simulink model "MoreElectricAircraftEMSHIL"  (R2023a)
settings: Solver=FixedStepAuto  StartTime=0.0  StopTime=350  RelTol=1e-3  EnableMultiTasking=on
PreLoadFcn:
  | Ts=100e-6;
InitFcn:
  | Ts=100e-6;
undefined symbols (not defined in the file): DiscIntNeverNeededParam, getfullname, IO682, Ion, Lithium
libraries: spsCurrentMeasurementLib x21, spsSeriesRLCBranchLib x19, spsVoltageMeasurementLib x19, speedgoatlib_IO682 x14, spsDiodeLib x10, spsControlledCurrentSourceLib x8, simulink x8, spsControlledVoltageSourceLib x7, spsIdealSwitchLib x6, spsThreePhaseParallelRLCLoadLib x1, spsPLL3phLib x1, spsThreePhaseVIMeasurementLib x1
(part 2 of 4)

== system MoreElectricAircraftEMSHIL/Hybrid Electric Aicraft System/Hybrid Electric Aicraft Plant/FC DC//DC Boost Converter ==
  VH* : Inport
  IL*(max) : Inport  Port=2
  Constant : Constant  Value=60
  DC/DC Boost Converter : Subsystem  mask(Average Value Boost DC/DC Converter){Inom=Inom, n=n, Tr=Tr, CL=CL}
      mask prompts: Inom "Full load current (A)"; n "Efficiency at Full and 10% load (%) [n1, n2]"; Tr "Response Time (s) (Voltage Regulator)"; CL "Load Capacitance (F)"
      mask help: This block implements an average-value DC/DC boost converter. Two inputs are provided for output voltage regulation and input current limitation
      mask init: same as MoreElectricAircraftEMSHIL/Hybrid Electric Aicraft System/Hybrid Electric Aicraft Plant/DC//DC Boost Converter/DC/DC Boost Converter
      mask DialogControl ParameterTabVar0 Prompt: Parameters
  DC/DC Buck Converter For DC bus precharge : Subsystem  mask(Average Value Buck DC/DC Converter){Inom=0.88*Inom, n=n, Tr=Tr, CL=CL}
      mask prompts: Inom "Full oad current (A)"; n "Efficiency @ Full and 10% load (%) [n1, n2]"; Tr "Response Time (s) (Voltage Regulator)"; CL "Load Capacitance (F)"
      mask help: This block implements an average-value DC/DC buck converter. Two inputs are provided for output voltage regulation and output current limitation
      mask init: same as MoreElectricAircraftEMSHIL/Hybrid Electric Aicraft System/Hybrid Electric Aicraft Plant/DC//DC Boost Converter/DC/DC Buck Converter For DC bus precharge
      mask DialogControl ParameterTabVar0 Prompt: Parameters
  +VH : PMIOPort  Side=Right
  +VL : PMIOPort  Port=2  Side=Left
  -VH : PMIOPort  Port=3  Side=Right
  -VL : PMIOPort  Port=4  Side=Left
  wires:
  [Iinbuck] -> DC/DC Boost Converter/3(Iinbuck)
  DC/DC Buck Converter For DC bus precharge/1(Iinbuck) -> [Iinbuck]
  Constant/1 -> DC/DC Buck Converter For DC bus precharge/1(VL*)
  VH*/1 -> DC/DC Boost Converter/1(VH*)
  IL*(max)/1 -> DC/DC Boost Converter/2(IL*(max)), DC/DC Buck Converter For DC bus precharge/2(IH*(max))
  connections:
  DC/DC Boost Converter/RConn2 -- -VH/RConn1 -- DC/DC Buck Converter For DC bus precharge/RConn2
  DC/DC Buck Converter For DC bus precharge/LConn2 -- -VL/RConn1 -- DC/DC Boost Converter/LConn2
  DC/DC Buck Converter For DC bus precharge/LConn1 -- +VL/RConn1 -- DC/DC Boost Converter/LConn1
  DC/DC Buck Converter For DC bus precharge/RConn1 -- +VH/RConn1 -- DC/DC Boost Converter/RConn1

== system MoreElectricAircraftEMSHIL/Hybrid Electric Aicraft System/Hybrid Electric Aicraft Plant/Fuel Cell Power Module (FCPM) ==
  Bus Selector : BusSelector  OutputSignals=Voltage,Current,Stack consumption (lpm) [Air(Yellow); Fuel(Magenta)],Flow Rate (lpm [Air(Yellow); Fuel(Magenta)]  OutputAsBus=on
  Contactors1 : Subsystem
  FCPM Controller : Subsystem
  Fuel Cell Stack : spsFuelCellStackLib/Fuel Cell Stack  PresetModel=No (User-Defined)  FcType=Proton Exchange Membrane (PEM)  Detailed=Detailed  Eoc="[52.5        52.46]"  NomVI="[250         41.15]"  EndVI="[320          39.2]"  Nc=65  n=50  TOp=45  AirFr=732  SuppPress="[1.16           1]"  Comp="[99.95           21            1]"  SignX=off  SignY=off  FlowRateH2=on  FlowRateAir=on  SystemTemp=off  SystemPH2=off  SystemPAir=off  FCDyn=on  FC_tau=1  Peak_O2=60  V_Under=2
      settings: LibrarySourceBlock=electricdrivelib/Extra Sources/Fuel Cell Stack
  Mux : Mux  Inputs=2
  Voltage Measurement : spsVoltageMeasurementLib/Voltage Measurement  PhasorSimulation=off  OutputType=Complex  PSBequivalent=0
  +VFC : PMIOPort  Side=Right
  -VFC : PMIOPort  Port=2  Side=Right
  Mesures : Outport  VectorParamsAs1DForOutWhenUnconnected=off
  Vfc : Outport  Port=2  VectorParamsAs1DForOutWhenUnconnected=off
  wires:
  FCPM Controller/3(H2Fr) -> Fuel Cell Stack/1
  FCPM Controller/2(AirFr) -> Fuel Cell Stack/2
  Fuel Cell Stack/1 -> FCPM Controller/1(IFC), Bus Selector/1
  FCPM Controller/1(IFCmax) -> Mux/1
  Bus Selector/1 -> Mux/2
  Mux/1 -> Mesures/1
  Voltage Measurement/1 -> Vfc/1
  connections:
  Contactors1/LConn1 -- Fuel Cell Stack/RConn1
  Voltage Measurement/LConn1 -- +VFC/RConn1 -- Contactors1/RConn1
  -VFC/RConn1 -- Fuel Cell Stack/RConn2 -- Voltage Measurement/LConn2

== system MoreElectricAircraftEMSHIL/Hybrid Electric Aicraft System/Hybrid Electric Aicraft Plant/Load Profile ==
  In1 : Inport
  1-D Lookup Table : Lookup_n-D  NumberOfTableDimensions=1  BreakpointsForDimension1="[0    20    30    35    40    45    50    60    70    90   125   130   140   160   170   180   190 210   220   230   235   245   250   260   270   300   310   320   330   340     350]"  Table="[0         0         0         0         0    5.8000    4.8000    4.8000   10.0000    9.4000  10.5000    5.0000    8.8000    7.0000    7.3000    2.5000    8.5000    7.5000    9.0000    8.9000 8.7000    0.7000    2.9000    2.3500    2.9000    2.9000    2.4000    2.9000    2.9000         0     0]"  InternalRulePriority=Speed  RndMeth=Simplest
  Aircraft Load(KVA) : Constant  Value=5.156351791530945
  Constant : Constant  Value=Ts
  Constant1 : Constant  Value=0
  Constant2 : Constant  Value=0.5
  Constant3 : Constant  Value=350
  Delay : Delay  DelayLength=1  InitialCondition=0
  Delay2 : Delay  DelayLength=1  InitialCondition=0
  Manual Load Control : Constant  Value=0
  Math Function : Math  Operator=mod
  Rate Transition : RateTransition  OutPortSampleTime=0.01
  Rate Transition1 : RateTransition
  Relational Operator : RelationalOperator  OutDataTypeStr=boolean  RndMeth=Simplest  InputSameDT=off
  Sum : Sum  Inputs=|++
  Sum1 : Sum  Inputs=|+-
  Switch : Switch  Criteria=u2 > Threshold  SaturateOnIntegerOverflow=off  InputSameDT=off
  Switch1 : Switch  Criteria=u2 > Threshold  Threshold=0.5  SaturateOnIntegerOverflow=off  InputSameDT=off
  Out1 : Outport
  wires:
  Constant1/1 -> Switch1/1
  Switch1/1 -> Math Function/1, Delay/1
  1-D Lookup Table/1 -> Switch/3
  Switch/1 -> Out1/1
  Constant/1 -> Sum/1
  Relational Operator/1 -> Switch1/2
  Sum/1 -> Switch1/3
  Constant2/1 -> Relational Operator/2
  Delay2/1 -> Sum1/2
  Aircraft Load(KVA)/1 -> Switch/1
  In1/1 -> Rate Transition/1
  Manual Load Control/1 -> Switch/2
  Delay/1 -> Sum/2
  Sum1/1 -> Rate Transition1/1
  Rate Transition/1 -> Delay2/1, Sum1/1
  Rate Transition1/1 -> Relational Operator/1
  Math Function/1 -> 1-D Lookup Table/1
  Constant3/1 -> Math Function/2

== system MoreElectricAircraftEMSHIL/Hybrid Electric Aicraft System/Hybrid Electric Aicraft Plant/Mesures 2 ==
  Current Measurement2 : spsCurrentMeasurementLib/Current Measurement  PhasorSimulation=off  OutputType=Complex  PSBequivalent=0
  Mux1 : Mux  Inputs=2
  Voltage Measurement2 : spsVoltageMeasurementLib/Voltage Measurement  PhasorSimulation=off  OutputType=Complex  PSBequivalent=0
  +M : PMIOPort  Side=Left
  O : PMIOPort  Port=2  Side=Right
  -M : PMIOPort  Port=3  Side=Left
  M : Outport  VectorParamsAs1DForOutWhenUnconnected=off
  wires:
  Voltage Measurement2/1 -> Mux1/2
  Current Measurement2/1 -> Mux1/1
  Mux1/1 -> M/1
  connections:
  +M/RConn1 -- Current Measurement2/LConn1
  -M/RConn1 -- Voltage Measurement2/LConn2
  Current Measurement2/RConn1 -- O/RConn1 -- Voltage Measurement2/LConn1

== system MoreElectricAircraftEMSHIL/Hybrid Electric Aicraft System/Hybrid Electric Aicraft Plant/Mesures1 ==
  Current Measurement2 : spsCurrentMeasurementLib/Current Measurement  PhasorSimulation=off  OutputType=Complex  PSBequivalent=0
  Mux1 : Mux  Inputs=2
  Voltage Measurement2 : spsVoltageMeasurementLib/Voltage Measurement  PhasorSimulation=off  OutputType=Complex  PSBequivalent=0
  +M : PMIOPort  Side=Left
  O : PMIOPort  Port=2  Side=Right
  -M : PMIOPort  Port=3  Side=Left
  M : Outport  VectorParamsAs1DForOutWhenUnconnected=off
  wires:
  Mux1/1 -> M/1
  Current Measurement2/1 -> Mux1/1
  Voltage Measurement2/1 -> Mux1/2
  connections:
  Voltage Measurement2/LConn1 -- O/RConn1 -- Current Measurement2/RConn1
  -M/RConn1 -- Voltage Measurement2/LConn2
  +M/RConn1 -- Current Measurement2/LConn1

== system MoreElectricAircraftEMSHIL/Hybrid Electric Aicraft System/Hybrid Electric Aicraft Plant/Protecting Resistor ==
  g : Inport
  Current Measurement : spsCurrentMeasurementLib/Current Measurement  PhasorSimulation=off  OutputType=Complex  PSBequivalent=0
  Ideal Switch : spsIdealSwitchLib/Ideal Switch  Ron=0.001  Lon=0  IC=0  Rs=10e3  Cs=inf  Measurements=off
  Mux : Mux  Inputs=2
  Series RLC Branch : spsSeriesRLCBranchLib/Series RLC Branch  LConnTagsString=__new0  RConnTagsString=__new0  BranchType=R  Resistance=6  Inductance=1e-3  SetiL0=off  InitialCurrent=0  Capacitance=1e-6  Setx0=off  InitialVoltage=0  Measurements=None
  Voltage Measurement : spsVoltageMeasurementLib/Voltage Measurement  PhasorSimulation=off  OutputType=Complex  PSBequivalent=0
  A : PMIOPort  Side=Right
  B : PMIOPort  Port=2  Side=Right
  Mesures : Outport  VectorParamsAs1DForOutWhenUnconnected=off
  wires:
  g/1 -> Ideal Switch/1
  Current Measurement/1 -> Mux/1
  Voltage Measurement/1 -> Mux/2
  Mux/1 -> Mesures/1
  connections:
  Series RLC Branch/LConn1 -- Ideal Switch/LConn1
  B/RConn1 -- Series RLC Branch/RConn1 -- Voltage Measurement/LConn2
  Current Measurement/RConn1 -- Ideal Switch/RConn1
  Current Measurement/LConn1 -- A/RConn1 -- Voltage Measurement/LConn1

== system MoreElectricAircraftEMSHIL/Hybrid Electric Aicraft System/Energy Management System/HIL/Plant Rx ==
  Bus Creator : BusCreator  Inputs=8
  "Decode v2 " : speedgoatlib_IO682/Decode v2   parMode=Standard  parLabel=[100 101 102 103 104 105 106 107]  parDataType=[1 1 1 1 1 1 1 1]  parResolution=[500 500 100 500 100 100 10 1]  parSyncMask=hex2dec('0x0')  parSyncValue=hex2dec('0x0')  parCustomDataType=Raw  parDataLSB=9  parDataMSB=31  parBitPosition=[9, 31]  parScaleBNR=1  parExponent=8  parMantissa=14  parTimeTags=off  parHoldLastVal=on  parStatus=off
      settings: SourceProductName=Simulink Real-Time: Speedgoat I/O Blockset
  Demux2 : Demux  Outputs=8
  Rate Transition4 : RateTransition  InitialCondition=1
  "Receive v3 " : speedgoatlib_IO682/Receive v3   parModuleId=1  parChannel=1  parMaxWords=50  parMinWords=1  parSampleTime=0.01
      settings: SourceProductName=Simulink Real-Time: Speedgoat I/O Blockset
  "Setup v3 " : speedgoatlib_IO682/Setup v3   parModuleId=1  parBoardVariant=IO682-4-4  parPciSlot=-1  parTimerCount=4000  parChannelMode=Manual  parInBitRate1=100000  parInBufferMode1=Individual  parInEnable1=on  parInParity1=on  parInInternalWrap1=off  parInBitRate2=100000  parInBufferMode2=Individual  parInEnable2=on  parInParity2=on  parInInternalWrap2=off  parInBitRate3=100000  parInBufferMode3=Individual  parInEnable3=on  parInParity3=on  parInInternalWrap3=off  parInBitRate4=100000  parInBufferMode4=Individual  parInEnable4=on  parInParity4=on  parInInternalWrap4=off  parInBitRate5=100000  parInBufferMode5=Individual  parInEnable5=on  parInParity5=on  parInInternalWrap5=off  parInBitRate6=100000  parInBufferMode6=Individual  parInEnable6=on  parInParity6=on  parInInternalWrap6=off  parInBitRate7=100000  parInBufferMode7=Individual  parInEnable7=on  parInParity7=on  parInInternalWrap7=off  parInBitRate8=100000  parInBufferMode8=Individual  parInEnable8=on  parInParity8=on  parInInternalWrap8=off  parInBitRate9=100000  parInBufferMode9=Individual  parInEnable9=on  parInParity9=on  parInInternalWrap9=off  parInBitRate10=100000  parInBufferMode10=Individual  parInEnable10=on  parInParity10=on  parInInternalWrap10=off  parInBitRate11=100000  parInBufferMode11=Individual  parInEnable11=on  parInParity11=on  parInInternalWrap11=off  parInBitRate12=100000  parInBufferMode12=Individual  parInEnable12=on  parInParity12=on  parInInternalWrap12=off  parInBitRate13=100000  parInBufferMode13=Individual  parInEnable13=on  parInParity13=on  parInInternalWrap13=off  parInBitRate14=100000  parInBufferMode14=Individual  parInEnable14=on  parInParity14=on  parInInternalWrap14=off  parInBitRate15=100000  parInBufferMode15=Individual  parInEnable15=on  parInParity15=on  parInInternalWrap15=off  parInBitRate16=100000  parInBufferMode16=Individual  parInEnable16=on  parInParity16=on  parInInternalWrap16=off  parOutBitRate1=100000  parOutParity1=Odd  parOutProtocolError1=None  parOutEnable1=on  parOutBitRate2=100000  parOutParity2=Odd  parOutProtocolError2=None  parOutEnable2=on  parOutBitRate3=100000  parOutParity3=Odd  parOutProtocolError3=None  parOutEnable3=on  parOutBitRate4=100000  parOutParity4=Odd  parOutProtocolError4=None  parOutEnable4=on  parOutBitRate5=100000  parOutParity5=Odd  parOutProtocolError5=None  parOutEnable5=on  parOutBitRate6=100000  parOutParity6=Odd  parOutProtocolError6=None  parOutEnable6=on  parOutBitRate7=100000  parOutParity7=Odd  parOutProtocolError7=None  parOutEnable7=on  parOutBitRate8=100000  parOutParity8=Odd  parOutProtocolError8=None  parOutEnable8=on  parOutBitRate9=100000  parOutParity9=Odd  parOutProtocolError9=None  parOutEnable9=on  parOutBitRate10=100000  parOutParity10=Odd  parOutProtocolError10=None  parOutEnable10=on  parOutBitRate11=100000  parOutParity11=Odd  parOutProtocolError11=None  parOutEnable11=on  parOutBitRate12=100000  parOutParity12=Odd  parOutProtocolError12=None  parOutEnable12=on  parOutBitRate13=100000  parOutParity13=Odd  parOutProtocolError13=None  parOutEnable13=on  parOutBitRate14=100000  parOutParity14=Odd  parOutProtocolError14=None  parOutEnable14=on  parOutBitRate15=100000  parOutParity15=Odd  parOutProtocolError15=None  parOutEnable15=on  parOutBitRate16=100000  parOutParity16=Odd  parOutProtocolError16=None  parOutEnable16=on  parChConfigFile=''  parScheduleMode=Manual  parScheduledMsgConfigFile=''  parHwDeviceId=hex2dec('0830')  parTimeSource=Internal timer  parChInConfig=[158 8 7 7 1;158 8 7 7 1;158 8 7 7 1;158 8 7 7 1]  parChOutConfig=[158 0 4 7;158 0 4 7;158 0 4 7;158 0 4 7]  parScheduledMessages=0  parIsSlrealtime=on
      settings: SourceProductName=Simulink Real-Time: Speedgoat I/O Blockset
  BusEMS : Outport
  wires:
  Rate Transition4/1 -> Demux2/1
  "Receive v3 "/1 -> "Decode v2 "/1
  "Decode v2 "/1 -> Rate Transition4/1
  Demux2/3 -> Bus Creator/3  "IBat_maxD"
  Demux2/7 -> Bus Creator/7  "Res_ON"
  Demux2/2 -> Bus Creator/2  "VDC1"
  Demux2/6 -> Bus Creator/6  "VBatt"
  Demux2/5 -> Bus Creator/5  "IBatt_maxC"
  Demux2/1 -> Bus Creator/1  "IFC_max"
  Demux2/8 -> Bus Creator/8  "Load_ON"
  Demux2/4 -> Bus Creator/4  "VDC2"
  Bus Creator/1 -> BusEMS/1

== system MoreElectricAircraftEMSHIL/Hybrid Electric Aicraft System/Energy Management System/HIL/Plant Tx ==
  BusPlant : Inport
  Bus Selector1 : BusSelector  OutputSignals=SOC (%),Current (A),Voltage (V)
  Bus Selector2 : BusSelector  OutputSignals=Current I,Voltage V,SOC %
  Bus Selector3 : BusSelector  OutputSignals=FuelCell,Battery,SC,IConvFCout,IConvBattout,Iinv,Vfc
  Encode v2 1 : speedgoatlib_IO682/Encode v2   parMode=Standard  parLabel=[300 301 302 303 304 305 306 307 310 311 312 313 314 315 316 317 320]  parDataType=[1 1 1 1 1 1 1 1 1 1 1 1 1 1 1 1 1]  parResolution=[300 100 300 300 100 700 100 100 100 100 100 300 100 100 100 100 100]  parBits=[19]  parSdi=[0]  parSsm=[-1]  parCustomDataType=Raw  parDataLSB=9  parDataMSB=31  parBitPosition=[9, 31]  parScaleBNR=1  parExponent=8  parMantissa=14  parEnSSM=off
      settings: SourceProductName=Simulink Real-Time: Speedgoat I/O Blockset
  Mux3 : Mux  Inputs=11
  Rate Transition : RateTransition
  Send v3 1 : speedgoatlib_IO682/Send v3   parModuleId=1  parChannel=2  parSampleTime=0.01
      settings: SourceProductName=Simulink Real-Time: Speedgoat I/O Blockset
  wires:
  Bus Selector2/1 -> Mux3/5  "<Current I>"
  Bus Selector1/1 -> Mux3/2  "<SOC (%)>"
  Bus Selector3/6 -> Mux3/10  "<Iinv>"
  Bus Selector3/4 -> Mux3/8  "<IConvFCout>"
  Bus Selector3/2 -> Bus Selector1/1  "<Battery>"
  Rate Transition/1 -> Send v3 1/1
  Bus Selector3/3 -> Bus Selector2/1  "<SC>"
  Bus Selector3/5 -> Mux3/9  "<IConvBattout>"
  Mux3/1 -> Encode v2 1/1
  Encode v2 1/1 -> Rate Transition/1
  Bus Selector3/1 -> Mux3/1  "<FuelCell>"
  BusPlant/1 -> Bus Selector3/1
  Bus Selector1/2 -> Mux3/3  "<Current (A)>"
  Bus Selector1/3 -> Mux3/4  "<Voltage (V)>"
  Bus Selector2/2 -> Mux3/6  "<Voltage V>"
  Bus Selector2/3 -> Mux3/7  "<SOC %>"
  Bus Selector3/7 -> Mux3/11  "<Vfc>"

== system MoreElectricAircraftEMSHIL/Hybrid Electric Aicraft System/Energy Management System/MIL/Battery DC//DC charge converter reference ==
  IBAT* : Inport
  Constant1 : Constant  Value=0
  Constant8 : Constant  Value=58
  Switch5 : Switch  Criteria=u2 > Threshold  SaturateOnIntegerOverflow=off  InputSameDT=off
  IBAT_maxC* : Outport  VectorParamsAs1DForOutWhenUnconnected=off
  VBAT* : Outport  Port=2  VectorParamsAs1DForOutWhenUnconnected=off
  wires:
  [EMSON] -> Switch5/2
  IBAT*/1 -> Switch5/1
  Constant1/1 -> Switch5/3
  Switch5/1 -> IBAT_maxC*/1
  Constant8/1 -> VBAT*/1

== system MoreElectricAircraftEMSHIL/Hybrid Electric Aicraft System/Energy Management System/MIL/Battery DC//DC discharge converter references  ==
  IBAT* : Inport
  Constant10 : Constant  Value=0
  Constant6 : Constant  Value=270
  Switch1 : Switch  Criteria=u2 > Threshold  SaturateOnIntegerOverflow=off  InputSameDT=off
  Switch10 : Switch  Criteria=u2 > Threshold  SaturateOnIntegerOverflow=off  InputSameDT=off
  IBAT_maxD* : Outport  VectorParamsAs1DForOutWhenUnconnected=off
  VDC2* : Outport  Port=2  VectorParamsAs1DForOutWhenUnconnected=off
  wires:
  Switch10/1 -> VDC2*/1
  [EMSON] -> Switch10/2
  Constant6/1 -> Switch10/3
  IBAT*/1 -> Switch1/1
  [Vdcref] -> Switch10/1
  [EMSON] -> Switch1/2
  Switch1/1 -> IBAT_maxD*/1
  Constant10/1 -> Switch1/3

== system MoreElectricAircraftEMSHIL/Hybrid Electric Aicraft System/Energy Management System/MIL/FC DC//DC converter references ==
  IFC* : Inport
  Add1 : Sum  Inputs=+-
  Constant11 : Constant  Value=212
  Constant22 : Constant  Value=270
  Constant3 : Constant  Value=15
  Constant4 : Constant  Value=297
  Constant7 : Constant  Value=250
  Fcn : Fcn  Expr=u(1)*(u(1)<u(2))+u(2)*(u(1)>=u(2))
  Mux6 : Mux  Inputs=2
  Relational Operator6 : RelationalOperator  Operator=<=  OutDataTypeStr=boolean  InputSameDT=off
  Switch : Switch  Criteria=u2 > Threshold  SaturateOnIntegerOverflow=off  InputSameDT=off
  Switch6 : Switch  Criteria=u2 > Threshold  SaturateOnIntegerOverflow=off  InputSameDT=off
  Switch9 : Switch  Criteria=u2 > Threshold  SaturateOnIntegerOverflow=off  InputSameDT=off
  filter : Subsystem
  IFC*max : Outport  VectorParamsAs1DForOutWhenUnconnected=off
  VDC1* : Outport  Port=2  VectorParamsAs1DForOutWhenUnconnected=off
  wires:
  [EMSON] -> Switch9/2
  Switch9/1 -> VDC1*/1
  Constant4/1 -> Switch9/1
  Constant22/1 -> Switch9/3
  Switch6/1 -> Switch/1
  Constant11/1 -> Relational Operator6/2, Switch6/3
  Relational Operator6/1 -> Switch6/2
  Constant7/1 -> Switch/3
  Constant3/1 -> Add1/2
  IFC*/1 -> Relational Operator6/1, Switch6/1
  Mux6/1 -> Fcn/1
  Fcn/1 -> filter/1(I)
  [EMSON] -> Switch/2
  Switch/1 -> Mux6/1
  filter/1(If) -> IFC*max/1
  Add1/1 -> Mux6/2
  [IFCAllow] -> Add1/1

== system MoreElectricAircraftEMSHIL/Hybrid Electric Aicraft System/Energy Management System/MIL/Load Disconnect ==
  SOC : Inport
  Vdc : Inport  Port=2
  Clock : Clock
  Constant1 : Constant  Value=0.1
  Constant18 : Constant  Value=0
  Constant19 : Constant  Value=0
  Constant2 : Constant  Value=270
  Constant5 : Constant
  Constant9 : Constant  Value=200
  Data Type Conversion2 : DataTypeConversion  SaturateOnIntegerOverflow=off  RndMeth=Floor
  Emergency_Landing : Constant
  Logical Operator : Logic  AllPortsSameDT=off  OutDataTypeStr=boolean
  Logical Operator3 : Logic  Inputs=3  AllPortsSameDT=off  OutDataTypeStr=boolean
  Relational Operator : RelationalOperator  OutDataTypeStr=boolean  InputSameDT=off
  Relational Operator1 : RelationalOperator  OutDataTypeStr=boolean  InputSameDT=off
  Relational Operator3 : RelationalOperator  Operator=<=  OutDataTypeStr=boolean  InputSameDT=off
  Relational Operator5 : RelationalOperator  Operator=<=  OutDataTypeStr=boolean  InputSameDT=off
  SOC_Low : Constant  Value=3
  Switch2 : Switch  Criteria=u2 > Threshold  SaturateOnIntegerOverflow=off  InputSameDT=off
  Switch7 : Switch  Criteria=u2 > Threshold  SaturateOnIntegerOverflow=off  InputSameDT=off
  Switch8 : Switch  Criteria=u2 > Threshold  SaturateOnIntegerOverflow=off  InputSameDT=off
  Unit Delay : UnitDelay  SampleTime=Ts  HasFrameUpgradeWarning=on
  Unit Delay4 : UnitDelay  InitialCondition=1  SampleTime=Ts  HasFrameUpgradeWarning=on
  LoadON : Outport  VectorParamsAs1DForOutWhenUnconnected=off
  tag scope: EMSON=global
  wires:
  Data Type Conversion2/1 -> LoadON/1  "Loadon"
  Relational Operator3/1 -> Switch8/2
  Constant18/1 -> Switch7/1
  Switch8/1 -> Switch2/3
  SOC_Low/1 -> Relational Operator5/2
  Switch7/1 -> Unit Delay4/1, Logical Operator3/1  "soc1"
  Unit Delay4/1 -> Switch7/3
  Unit Delay/1 -> Switch8/3
  SOC/1 -> Relational Operator5/1
  Logical Operator3/1 -> Data Type Conversion2/1
  Constant19/1 -> Switch8/1
  Constant9/1 -> Relational Operator3/2
  Relational Operator/1 -> Switch2/2
  Constant5/1 -> Switch2/1
  Constant2/1 -> Relational Operator/2
  Switch2/1 -> [EMSON], Unit Delay/1, Logical Operator3/2
  Vdc/1 -> Relational Operator/1, Relational Operator3/1
  Relational Operator5/1 -> Logical Operator/2  "Battery Health"
  Clock/1 -> Relational Operator1/1
  Constant1/1 -> Relational Operator1/2
  Relational Operator1/1 -> Logical Operator/1
  Logical Operator/1 -> Switch7/2
  Emergency_Landing/1 -> Logical Operator3/3

== system MoreElectricAircraftEMSHIL/Hybrid Electric Aicraft System/Energy Management System/MIL/Protecting resistor connect ==
  Vdc : Inport
  Constant12 : Constant  Value=290
  Constant13 : Constant
  Constant14 : Constant  Value=285
  Constant15 : Constant  Value=0
  Data Type Conversion1 : DataTypeConversion  SaturateOnIntegerOverflow=off  RndMeth=Floor
  Relational Operator1 : RelationalOperator  OutDataTypeStr=boolean  InputSameDT=off
  Relational Operator2 : RelationalOperator  Operator=<=  OutDataTypeStr=boolean  InputSameDT=off
  Switch3 : Switch  Criteria=u2 > Threshold  SaturateOnIntegerOverflow=off  InputSameDT=off
  Switch4 : Switch  Criteria=u2 > Threshold  SaturateOnIntegerOverflow=off  InputSameDT=off
  Unit Delay1 : UnitDelay  SampleTime=Ts  HasFrameUpgradeWarning=on
  ResON : Outport  VectorParamsAs1DForOutWhenUnconnected=off
  wires:
  Unit Delay1/1 -> Switch4/3
  Vdc/1 -> Relational Operator1/1, Relational Operator2/1
  Switch4/1 -> Switch3/3
  Switch3/1 -> Data Type Conversion1/1, Unit Delay1/1
  Relational Operator1/1 -> Switch3/2
  Relational Operator2/1 -> Switch4/2
  Data Type Conversion1/1 -> ResON/1
  Constant15/1 -> Switch4/1
  Constant13/1 -> Switch3/1
  Constant14/1 -> Relational Operator2/2
  Constant12/1 -> Relational Operator1/2

== system MoreElectricAircraftEMSHIL/Hybrid Electric Aicraft System/Energy Management System/MIL/Subsystem ==
  note: Max DC bus voltage
  note: Min DC bus voltage
  Pload : Inport
  SOC : Inport  Port=2
  Constant1 : Constant  Value=260
  Constant2 : Constant  Value=285
  Constant20 : Constant  Value=270
  Constant21 : Constant  Value=60
  Discrete PI Controller1 : Subsystem  DialogController=POWERSYS.PowerSysDialog  mask(Discrete PI Controller){Kp=10, Ki=10, Par_Limits=[140 0], Init=0, Ts=Ts}
      mask prompts: Kp "Proportional gain (Kp):"; Ki "Integral gain (Ki):"; Par_Limits "Output limits: [ Upper   Lower ]"; Init "Output initial value:"; Ts "Sample time:"
      mask help: This block implements a discrete PI controller.
      mask init:
      | UpperLimit=Par_Limits(1);
      | LowerLimit=Par_Limits(2);
      | power_initmask();
      mask Help: This block is part of a subset of blocks in the Extras library that does not have documentation associated with it, other than the block mask description.
      mask Display: disp('PI');
  Discrete PI Controller2 : Subsystem  DialogController=POWERSYS.PowerSysDialog  mask(Discrete PI Controller){Kp=50000, Ki=5000, Par_Limits=[3400 -1500], Init=0, Ts=200e-3}
      mask prompts: Kp "Proportional gain (Kp):"; Ki "Integral gain (Ki):"; Par_Limits "Output limits: [ Upper   Lower ]"; Init "Output initial value:"; Ts "Sample time:"
      mask help: This block implements a discrete PI controller.
      mask init:
      | UpperLimit=Par_Limits(1);
      | LowerLimit=Par_Limits(2);
      | power_initmask();
      mask Help: This block is part of a subset of blocks in the Extras library that does not have documentation associated with it, other than the block mask description.
      mask Display: disp('PI');
  Discrete PI Controller3 : Subsystem  DialogController=POWERSYS.PowerSysDialog  mask(Discrete PI Controller){Kp=10, Ki=10, Par_Limits=[0 -100], Init=0, Ts=Ts}
      mask prompts: Kp "Proportional gain (Kp):"; Ki "Integral gain (Ki):"; Par_Limits "Output limits: [ Upper   Lower ]"; Init "Output initial value:"; Ts "Sample time:"
      mask help: This block implements a discrete PI controller.
      mask init:
      | UpperLimit=Par_Limits(1);
      | LowerLimit=Par_Limits(2);
      | power_initmask();
      mask Help: This block is part of a subset of blocks in the Extras library that does not have documentation associated with it, other than the block mask description.
      mask Display: disp('PI');
  Discrete PI Controller4 : Subsystem  DialogController=POWERSYS.PowerSysDialog  mask(Discrete PI Controller){Kp=10, Ki=10, Par_Limits=[80 -20], Init=0, Ts=Ts}
      mask prompts: Kp "Proportional gain (Kp):"; Ki "Integral gain (Ki):"; Par_Limits "Output limits: [ Upper   Lower ]"; Init "Output initial value:"; Ts "Sample time:"
      mask help: This block implements a discrete PI controller.
      mask init:
      | UpperLimit=Par_Limits(1);
      | LowerLimit=Par_Limits(2);
      | power_initmask();
      mask Help: This block is part of a subset of blocks in the Extras library that does not have documentation associated with it, other than the block mask description.
      mask Display: disp('PI');
  Divide : Product  Inputs=*/
  Gain : Gain  Gain=-1
  Gain2 : Gain  Gain=1/0.85
  Saturation : Saturate  UpperLimit=inf  LowerLimit=0.01
  Saturation1 : Saturate  UpperLimit=80  LowerLimit=0
  Saturation2 : Saturate  UpperLimit=20  LowerLimit=0
  Saturation3 : Saturate  UpperLimit=8800  LowerLimit=850
  Saturation4 : Saturate  UpperLimit=250  LowerLimit=20
  Sum : Sum  Inputs=|+-
  Sum1 : Sum  Inputs=|-+
  Sum2 : Sum  Inputs=|-+
  Sum3 : Sum  Inputs=|+-
  Sum4 : Sum  Inputs=|++
  Sum5 : Sum  Inputs=|+-
  Sum6 : Sum  Inputs=|++
  filter2 : Subsystem
  IFC* : Outport  VectorParamsAs1DForOutWhenUnconnected=off
  IBATD* : Outport  Port=2  VectorParamsAs1DForOutWhenUnconnected=off
  IBATC* : Outport  Port=3  VectorParamsAs1DForOutWhenUnconnected=off
  tag scope: Vdcref=scoped
  wires:
  Divide/1 -> Sum4/1
  Discrete PI Controller1/1(Out) -> Sum4/2
  filter2/1(If) -> IBATC*/1
  Constant20/1 -> Sum/1, [Vdcref]
  SOC/1 -> Sum1/2
  Saturation3/1 -> Gain2/1
  Saturation/1 -> Divide/2
  Saturation1/1 -> IBATD*/1
  Constant1/1 -> Sum3/1
  Discrete PI Controller2/1(Out) -> Sum2/1
  Sum5/1 -> Discrete PI Controller3/1(Error)
  Sum4/1 -> Sum6/1
  Constant21/1 -> Sum1/1
  Pload/1 -> Sum2/2
  Gain2/1 -> Divide/1
  Sum6/1 -> Saturation4/1
  Saturation4/1 -> IFC*/1
  Constant2/1 -> Sum5/1
  Sum3/1 -> Discrete PI Controller1/1(Error)
  Gain/1 -> Saturation2/1
  Discrete PI Controller4/1(Out) -> Saturation1/1, Gain/1
  Sum2/1 -> Saturation3/1
  Sum1/1 -> Discrete PI Controller2/1(Error)
  Saturation2/1 -> filter2/1(I)
  [Vdc] -> Sum5/2
  [Vdc] -> Sum/2
  Discrete PI Controller3/1(Out) -> Sum6/2
  [Vdc] -> Sum3/2
  [S_Vfc] -> Saturation/1
  Sum/1 -> Discrete PI Controller4/1(Error)

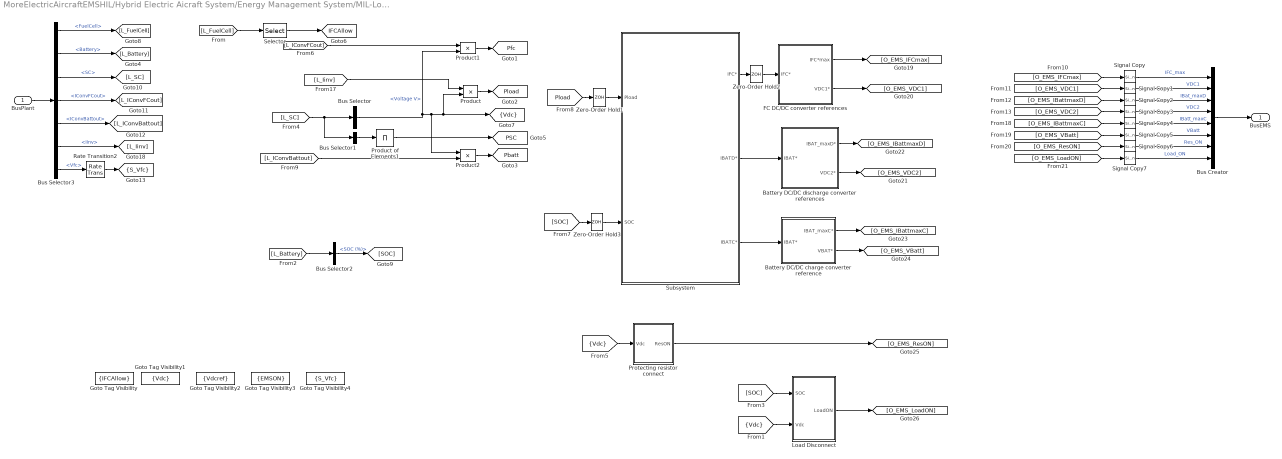
== system MoreElectricAircraftEMSHIL/Hybrid Electric Aicraft System/Energy Management System/MIL-Loopback/EMS ==
  BusPlant : Inport
  Battery DC/DC charge converter reference : Subsystem
  "Battery DC/DC discharge converter references " : Subsystem
  Bus Creator : BusCreator  Inputs=8
  Bus Selector : BusSelector  OutputSignals=Voltage V
  Bus Selector1 : BusSelector  OutputSignals=Current I,Voltage V  OutputAsBus=on
  Bus Selector2 : BusSelector  OutputSignals=SOC (%)
  Bus Selector3 : BusSelector  OutputSignals=FuelCell,Battery,SC,IConvFCout,IConvBattout,Iinv,Vfc
  FC DC/DC converter references : Subsystem
  Goto Tag Visibility : GotoTagVisibility  GotoTag=IFCAllow
  Goto Tag Visibility1 : GotoTagVisibility  GotoTag=Vdc
  Goto Tag Visibility2 : GotoTagVisibility  GotoTag=Vdcref
  Goto Tag Visibility3 : GotoTagVisibility  GotoTag=EMSON
  Goto Tag Visibility4 : GotoTagVisibility  GotoTag=S_Vfc
  Load Disconnect : Subsystem
  Product : Product  RndMeth=Zero
  Product of Elements1 : Product  Inputs=*
  Product1 : Product  RndMeth=Zero
  Product2 : Product  RndMeth=Zero
  Protecting resistor connect : Subsystem
  Rate Transition2 : RateTransition  InitialCondition=1
  Selector : Selector  InputPortWidth=7  IndexOptions=Index vector (dialog)  Indices=1  OutputSizes=1
  Signal Copy{,1..7} (8 alike) : SignalConversion  OverrideOpt=off
  Subsystem : Subsystem
  Zero-Order Hold1 : ZeroOrderHold  SampleTime=200e-3
  Zero-Order Hold2 : ZeroOrderHold  SampleTime=200e-3
  Zero-Order Hold3 : ZeroOrderHold  SampleTime=200e-3
  BusEMS : Outport  VectorParamsAs1DForOutWhenUnconnected=off
  tag scope: IFCAllow=global, PSC=global, Pbatt=global, Pfc=global, Pload=global, S_Vfc=scoped, Vdc=scoped
  wires:
  Bus Selector/1 -> Product1/2, Product2/1, Product/2, [Vdc]  "<Voltage V>"
  [L_IConvFCout] -> Product1/1
  [L_IConvBattout] -> Product2/2
  [L_Iinv] -> Product/1
  [L_SC] -> Bus Selector/1, Bus Selector1/1
  Product/1 -> [Pload]
  Product1/1 -> [Pfc]
  Product2/1 -> [Pbatt]
  Bus Selector1/1 -> Product of Elements1/1
  Product of Elements1/1 -> [PSC]
  Selector/1 -> [IFCAllow]
  [L_Battery] -> Bus Selector2/1
  Bus Selector2/1 -> [SOC]  "<SOC (%)>"
  [SOC] -> Load Disconnect/1(SOC)
  [Vdc] -> Load Disconnect/2(Vdc)
  [Vdc] -> Protecting resistor connect/1(Vdc)
  Subsystem/1(IFC*) -> Zero-Order Hold2/1
  [Pload] -> Zero-Order Hold1/1
  [SOC] -> Zero-Order Hold3/1
  Zero-Order Hold2/1 -> FC DC/DC converter references/1(IFC*)
  Subsystem/2(IBATD*) -> "Battery DC/DC discharge converter references "/1(IBAT*)
  Subsystem/3(IBATC*) -> Battery DC/DC charge converter reference/1(IBAT*)
  Zero-Order Hold1/1 -> Subsystem/1(Pload)
  Zero-Order Hold3/1 -> Subsystem/2(SOC)
  FC DC/DC converter references/1(IFC*max) -> [O_EMS_IFCmax]
  FC DC/DC converter references/2(VDC1*) -> [O_EMS_VDC1]
  "Battery DC/DC discharge converter references "/1(IBAT_maxD*) -> [O_EMS_IBattmaxD]
  "Battery DC/DC discharge converter references "/2(VDC2*) -> [O_EMS_VDC2]
  Battery DC/DC charge converter reference/1(IBAT_maxC*) -> [O_EMS_IBattmaxC]
  Battery DC/DC charge converter reference/2(VBAT*) -> [O_EMS_VBatt]
  Protecting resistor connect/1(ResON) -> [O_EMS_ResON]
  Load Disconnect/1(LoadON) -> [O_EMS_LoadON]
  BusPlant/1 -> Bus Selector3/1
  Bus Selector3/1 -> [L_FuelCell]  "<FuelCell>"
  Bus Selector3/2 -> [L_Battery]  "<Battery>"
  Bus Selector3/3 -> [L_SC]  "<SC>"
  Bus Selector3/4 -> [L_IConvFCout]  "<IConvFCout>"
  Bus Selector3/5 -> [L_IConvBattout]  "<IConvBattout>"
  Bus Selector3/6 -> [L_Iinv]  "<Iinv>"
  [L_FuelCell] -> Selector/1
  [O_EMS_IFCmax] -> Signal Copy/1
  [O_EMS_VDC1] -> Signal Copy1/1
  [O_EMS_IBattmaxD] -> Signal Copy2/1
  [O_EMS_VDC2] -> Signal Copy3/1
  [O_EMS_IBattmaxC] -> Signal Copy4/1
  [O_EMS_VBatt] -> Signal Copy5/1
  [O_EMS_ResON] -> Signal Copy6/1
  [O_EMS_LoadON] -> Signal Copy7/1
  Signal Copy1/1 -> Bus Creator/2  "VDC1"
  Signal Copy2/1 -> Bus Creator/3  "IBat_maxD"
  Signal Copy3/1 -> Bus Creator/4  "VDC2"
  Signal Copy4/1 -> Bus Creator/5  "IBatt_maxC"
  Signal Copy5/1 -> Bus Creator/6  "VBatt"
  Signal Copy6/1 -> Bus Creator/7  "Res_ON"
  Signal Copy7/1 -> Bus Creator/8  "Load_ON"
  Signal Copy/1 -> Bus Creator/1  "IFC_max"
  Bus Creator/1 -> BusEMS/1
  Bus Selector3/7 -> Rate Transition2/1  "<Vfc>"
  Rate Transition2/1 -> [S_Vfc]

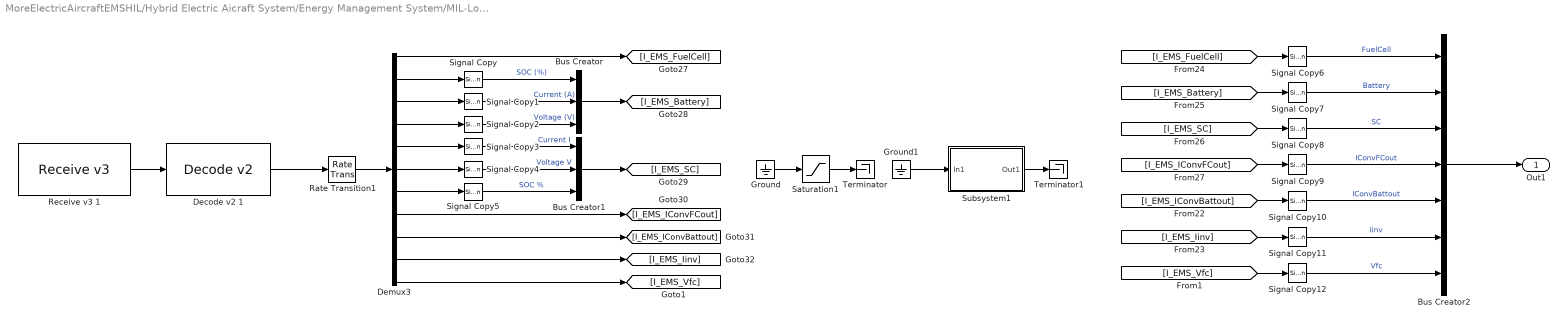
== system MoreElectricAircraftEMSHIL/Hybrid Electric Aicraft System/Energy Management System/MIL-Loopback/EMS Rx ==
  Bus Creator : BusCreator  Inputs=3
  Bus Creator1 : BusCreator  Inputs=3
  Bus Creator2 : BusCreator  Inputs=7
  Decode v2 1 : speedgoatlib_IO682/Decode v2   parMode=Standard  parLabel=[300 301 302 303 304 305 306 307 310 311 312 313 314 315 316 317 320]  parDataType=[1 1 1 1 1 1 1 1 1 1 1 1 1 1 1 1 1]  parResolution=[300 100 300 300 100 700 100 100 100 100 100 300 100 100 100 100 100]  parSyncMask=hex2dec('0x0')  parSyncValue=hex2dec('0x0')  parCustomDataType=Raw  parDataLSB=9  parDataMSB=31  parBitPosition=[9, 31]  parScaleBNR=1  parExponent=8  parMantissa=14  parTimeTags=off  parHoldLastVal=on  parStatus=off
      settings: SourceProductName=Simulink Real-Time: Speedgoat I/O Blockset
  Demux3 : Demux  Outputs=11
  Ground : Ground
  Ground1 : Ground
  Rate Transition1 : RateTransition  InitialCondition=1
  Receive v3 1 : speedgoatlib_IO682/Receive v3   parModuleId=1  parChannel=2  parMaxWords=100  parMinWords=1  parSampleTime=0.01
      settings: SourceProductName=Simulink Real-Time: Speedgoat I/O Blockset
  Saturation1 : Saturate  UpperLimit=1000000000  LowerLimit=269
  Signal Copy{,1..12} (13 alike) : SignalConversion  OverrideOpt=off
  Subsystem1 : Subsystem
  Terminator : Terminator
  Terminator1 : Terminator
  Out1 : Outport
  wires:
  Subsystem1/1(Out1) -> Terminator1/1
  Ground/1 -> Saturation1/1
  Demux3/2 -> Signal Copy/1
  Rate Transition1/1 -> Demux3/1
  Demux3/1 -> [I_EMS_FuelCell]
  Signal Copy1/1 -> Bus Creator/2  "Current (A)"
  Signal Copy5/1 -> Bus Creator1/3  "SOC %"
  Bus Creator1/1 -> [I_EMS_SC]
  Demux3/9 -> [I_EMS_IConvBattout]
  Demux3/5 -> Signal Copy3/1
  Bus Creator/1 -> [I_EMS_Battery]
  Signal Copy4/1 -> Bus Creator1/2  "Voltage V"
  Demux3/7 -> Signal Copy5/1
  Signal Copy3/1 -> Bus Creator1/1  "Current I"
  Saturation1/1 -> Terminator/1
  Ground1/1 -> Subsystem1/1(In1)
  Demux3/6 -> Signal Copy4/1
  Demux3/4 -> Signal Copy2/1
  Decode v2 1/1 -> Rate Transition1/1
  Signal Copy2/1 -> Bus Creator/3  "Voltage (V)"
  Demux3/10 -> [I_EMS_Iinv]
  Demux3/3 -> Signal Copy1/1
  Receive v3 1/1 -> Decode v2 1/1
  Signal Copy/1 -> Bus Creator/1  "SOC (%)"
  Demux3/8 -> [I_EMS_IConvFCout]
  Bus Creator2/1 -> Out1/1
  Signal Copy9/1 -> Bus Creator2/4  "IConvFCout"
  Signal Copy8/1 -> Bus Creator2/3  "SC"
  Signal Copy10/1 -> Bus Creator2/5  "IConvBattout"
  [I_EMS_Battery] -> Signal Copy7/1
  Signal Copy11/1 -> Bus Creator2/6  "Iinv"
  [I_EMS_Iinv] -> Signal Copy11/1
  [I_EMS_SC] -> Signal Copy8/1
  [I_EMS_IConvBattout] -> Signal Copy10/1
  Signal Copy6/1 -> Bus Creator2/1  "FuelCell"
  Signal Copy7/1 -> Bus Creator2/2  "Battery"
  [I_EMS_IConvFCout] -> Signal Copy9/1
  [I_EMS_FuelCell] -> Signal Copy6/1
  Demux3/11 -> [I_EMS_Vfc]
  [I_EMS_Vfc] -> Signal Copy12/1
  Signal Copy12/1 -> Bus Creator2/7  "Vfc"

== system MoreElectricAircraftEMSHIL/Hybrid Electric Aicraft System/Energy Management System/MIL-Loopback/EMS Tx ==
  IFC*max1 : Inport
  Bus Selector3 : BusSelector  OutputSignals=IFC_max,VDC1,IBat_maxD,VDC2,IBatt_maxC,VBatt,Res_ON,Load_ON
  "Encode v2 " : speedgoatlib_IO682/Encode v2   parMode=Standard  parLabel=[100 101 102 103 104 105 106 107]  parDataType=[1 1 1 1 1 1 1 1]  parResolution=[500 500 100 500 100 100 10 1]  parBits=[19]  parSdi=[0]  parSsm=[-1]  parCustomDataType=Raw  parDataLSB=9  parDataMSB=31  parBitPosition=[9, 31]  parScaleBNR=1  parExponent=8  parMantissa=14  parEnSSM=off
      settings: SourceProductName=Simulink Real-Time: Speedgoat I/O Blockset
  Mux2 : Mux  Inputs=8
  Rate Transition3 : RateTransition
  "Send v3 " : speedgoatlib_IO682/Send v3   parModuleId=1  parChannel=1  parSampleTime=0.01
      settings: SourceProductName=Simulink Real-Time: Speedgoat I/O Blockset
  "Setup v3 " : speedgoatlib_IO682/Setup v3   parModuleId=1  parBoardVariant=IO682-4-4  parPciSlot=-1  parTimerCount=4000  parChannelMode=Manual  parInBitRate1=100000  parInBufferMode1=Individual  parInEnable1=on  parInParity1=on  parInInternalWrap1=off  parInBitRate2=100000  parInBufferMode2=Individual  parInEnable2=on  parInParity2=on  parInInternalWrap2=off  parInBitRate3=100000  parInBufferMode3=Individual  parInEnable3=on  parInParity3=on  parInInternalWrap3=off  parInBitRate4=100000  parInBufferMode4=Individual  parInEnable4=on  parInParity4=on  parInInternalWrap4=off  parInBitRate5=100000  parInBufferMode5=Individual  parInEnable5=on  parInParity5=on  parInInternalWrap5=off  parInBitRate6=100000  parInBufferMode6=Individual  parInEnable6=on  parInParity6=on  parInInternalWrap6=off  parInBitRate7=100000  parInBufferMode7=Individual  parInEnable7=on  parInParity7=on  parInInternalWrap7=off  parInBitRate8=100000  parInBufferMode8=Individual  parInEnable8=on  parInParity8=on  parInInternalWrap8=off  parInBitRate9=100000  parInBufferMode9=Individual  parInEnable9=on  parInParity9=on  parInInternalWrap9=off  parInBitRate10=100000  parInBufferMode10=Individual  parInEnable10=on  parInParity10=on  parInInternalWrap10=off  parInBitRate11=100000  parInBufferMode11=Individual  parInEnable11=on  parInParity11=on  parInInternalWrap11=off  parInBitRate12=100000  parInBufferMode12=Individual  parInEnable12=on  parInParity12=on  parInInternalWrap12=off  parInBitRate13=100000  parInBufferMode13=Individual  parInEnable13=on  parInParity13=on  parInInternalWrap13=off  parInBitRate14=100000  parInBufferMode14=Individual  parInEnable14=on  parInParity14=on  parInInternalWrap14=off  parInBitRate15=100000  parInBufferMode15=Individual  parInEnable15=on  parInParity15=on  parInInternalWrap15=off  parInBitRate16=100000  parInBufferMode16=Individual  parInEnable16=on  parInParity16=on  parInInternalWrap16=off  parOutBitRate1=100000  parOutParity1=Odd  parOutProtocolError1=None  parOutEnable1=on  parOutBitRate2=100000  parOutParity2=Odd  parOutProtocolError2=None  parOutEnable2=on  parOutBitRate3=100000  parOutParity3=Odd  parOutProtocolError3=None  parOutEnable3=on  parOutBitRate4=100000  parOutParity4=Odd  parOutProtocolError4=None  parOutEnable4=on  parOutBitRate5=100000  parOutParity5=Odd  parOutProtocolError5=None  parOutEnable5=on  parOutBitRate6=100000  parOutParity6=Odd  parOutProtocolError6=None  parOutEnable6=on  parOutBitRate7=100000  parOutParity7=Odd  parOutProtocolError7=None  parOutEnable7=on  parOutBitRate8=100000  parOutParity8=Odd  parOutProtocolError8=None  parOutEnable8=on  parOutBitRate9=100000  parOutParity9=Odd  parOutProtocolError9=None  parOutEnable9=on  parOutBitRate10=100000  parOutParity10=Odd  parOutProtocolError10=None  parOutEnable10=on  parOutBitRate11=100000  parOutParity11=Odd  parOutProtocolError11=None  parOutEnable11=on  parOutBitRate12=100000  parOutParity12=Odd  parOutProtocolError12=None  parOutEnable12=on  parOutBitRate13=100000  parOutParity13=Odd  parOutProtocolError13=None  parOutEnable13=on  parOutBitRate14=100000  parOutParity14=Odd  parOutProtocolError14=None  parOutEnable14=on  parOutBitRate15=100000  parOutParity15=Odd  parOutProtocolError15=None  parOutEnable15=on  parOutBitRate16=100000  parOutParity16=Odd  parOutProtocolError16=None  parOutEnable16=on  parChConfigFile=''  parScheduleMode=Manual  parScheduledMsgConfigFile=''  parHwDeviceId=hex2dec('0830')  parTimeSource=Internal timer  parChInConfig=[158 8 7 7 1;158 8 7 7 1;158 8 7 7 1;158 8 7 7 1]  parChOutConfig=[158 0 4 7;158 0 4 7;158 0 4 7;158 0 4 7]  parScheduledMessages=0  parIsSlrealtime=on
      settings: SourceProductName=Simulink Real-Time: Speedgoat I/O Blockset
  wires:
  "Encode v2 "/1 -> Rate Transition3/1
  Mux2/1 -> "Encode v2 "/1
  Rate Transition3/1 -> "Send v3 "/1
  IFC*max1/1 -> Bus Selector3/1
  Bus Selector3/1 -> Mux2/1  "<IFC_max>"
  Bus Selector3/2 -> Mux2/2  "<VDC1>"
  Bus Selector3/3 -> Mux2/3  "<IBat_maxD>"
  Bus Selector3/4 -> Mux2/4  "<VDC2>"
  Bus Selector3/5 -> Mux2/5  "<IBatt_maxC>"
  Bus Selector3/6 -> Mux2/6  "<VBatt>"
  Bus Selector3/7 -> Mux2/7  "<Res_ON>"
  Bus Selector3/8 -> Mux2/8  "<Load_ON>"

== system MoreElectricAircraftEMSHIL/Hybrid Electric Aicraft System/Energy Management System/MIL-Loopback/Plant Rx ==
  Bus Creator : BusCreator  Inputs=8
  "Decode v2 " : speedgoatlib_IO682/Decode v2   parMode=Standard  parLabel=[100 101 102 103 104 105 106 107]  parDataType=[1 1 1 1 1 1 1 1]  parResolution=[500 500 100 500 100 100 10 1]  parSyncMask=hex2dec('0x0')  parSyncValue=hex2dec('0x0')  parCustomDataType=Raw  parDataLSB=9  parDataMSB=31  parBitPosition=[9, 31]  parScaleBNR=1  parExponent=8  parMantissa=14  parTimeTags=off  parHoldLastVal=on  parStatus=off
      settings: SourceProductName=Simulink Real-Time: Speedgoat I/O Blockset
  Demux2 : Demux  Outputs=8
  Rate Transition4 : RateTransition  InitialCondition=1
  "Receive v3 " : speedgoatlib_IO682/Receive v3   parModuleId=1  parChannel=1  parMaxWords=50  parMinWords=1  parSampleTime=0.01
      settings: SourceProductName=Simulink Real-Time: Speedgoat I/O Blockset
  BusEMS : Outport
  wires:
  Rate Transition4/1 -> Demux2/1
  "Receive v3 "/1 -> "Decode v2 "/1
  "Decode v2 "/1 -> Rate Transition4/1
  Demux2/3 -> Bus Creator/3  "IBat_maxD"
  Demux2/7 -> Bus Creator/7  "Res_ON"
  Demux2/2 -> Bus Creator/2  "VDC1"
  Demux2/6 -> Bus Creator/6  "VBatt"
  Demux2/5 -> Bus Creator/5  "IBatt_maxC"
  Demux2/1 -> Bus Creator/1  "IFC_max"
  Demux2/8 -> Bus Creator/8  "Load_ON"
  Demux2/4 -> Bus Creator/4  "VDC2"
  Bus Creator/1 -> BusEMS/1

== system MoreElectricAircraftEMSHIL/Hybrid Electric Aicraft System/Energy Management System/MIL-Loopback/Plant Tx ==
  BusPlant : Inport
  Bus Selector1 : BusSelector  OutputSignals=SOC (%),Current (A),Voltage (V)
  Bus Selector2 : BusSelector  OutputSignals=Current I,Voltage V,SOC %
  Bus Selector3 : BusSelector  OutputSignals=FuelCell,Battery,SC,IConvFCout,IConvBattout,Iinv,Vfc
  Encode v2 1 : speedgoatlib_IO682/Encode v2   parMode=Standard  parLabel=[300 301 302 303 304 305 306 307 310 311 312 313 314 315 316 317 320]  parDataType=[1 1 1 1 1 1 1 1 1 1 1 1 1 1 1 1 1]  parResolution=[300 100 300 300 100 700 100 100 100 100 100 300 100 100 100 100 100]  parBits=[19]  parSdi=[0]  parSsm=[-1]  parCustomDataType=Raw  parDataLSB=9  parDataMSB=31  parBitPosition=[9, 31]  parScaleBNR=1  parExponent=8  parMantissa=14  parEnSSM=off
      settings: SourceProductName=Simulink Real-Time: Speedgoat I/O Blockset
  Mux3 : Mux  Inputs=11
  Rate Transition : RateTransition
  Send v3 1 : speedgoatlib_IO682/Send v3   parModuleId=1  parChannel=2  parSampleTime=0.01
      settings: SourceProductName=Simulink Real-Time: Speedgoat I/O Blockset
  wires:
  Bus Selector2/1 -> Mux3/5  "<Current I>"
  Bus Selector1/1 -> Mux3/2  "<SOC (%)>"
  Bus Selector3/6 -> Mux3/10  "<Iinv>"
  Bus Selector3/4 -> Mux3/8  "<IConvFCout>"
  Bus Selector3/2 -> Bus Selector1/1  "<Battery>"
  Rate Transition/1 -> Send v3 1/1
  Bus Selector3/3 -> Bus Selector2/1  "<SC>"
  Bus Selector3/5 -> Mux3/9  "<IConvBattout>"
  Mux3/1 -> Encode v2 1/1
  Encode v2 1/1 -> Rate Transition/1
  Bus Selector3/1 -> Mux3/1  "<FuelCell>"
  BusPlant/1 -> Bus Selector3/1
  Bus Selector1/2 -> Mux3/3  "<Current (A)>"
  Bus Selector1/3 -> Mux3/4  "<Voltage (V)>"
  Bus Selector2/2 -> Mux3/6  "<Voltage V>"
  Bus Selector2/3 -> Mux3/7  "<SOC %>"
  Bus Selector3/7 -> Mux3/11  "<Vfc>"

== system MoreElectricAircraftEMSHIL/Hybrid Electric Aicraft System/Hybrid Electric Aicraft Plant/3-phase AC load/Dynamic Impedance ==
  S : Inport
  pf : Inport  Port=2
  Fcn3 : Fcn  Expr=(sqrt(u(2)^2-u(1)^2))
  Fcn5 : Fcn  Expr=u(1)*u(2)
  Gain1 : Gain  Gain=2e3
  Gain3 : Gain  Gain=2e3
  Impedance Calculation : Subsystem
  Mux1 : Mux  Inputs=2
  Mux3 : Mux  Inputs=2
  Real-Imag to Complex1 : RealImagToComplex
  Z : Outport  VectorParamsAs1DForOutWhenUnconnected=off
  wires:
  Gain1/1 -> Real-Imag to Complex1/1
  Gain3/1 -> Real-Imag to Complex1/2
  Real-Imag to Complex1/1 -> Impedance Calculation/1(S)
  Impedance Calculation/1(Z) -> Z/1
  Mux1/1 -> Fcn5/1
  pf/1 -> Mux1/2
  Fcn5/1 -> Mux3/1, Gain1/1
  Mux3/1 -> Fcn3/1
  Fcn3/1 -> Gain3/1
  S/1 -> Mux1/1, Mux3/2

== system MoreElectricAircraftEMSHIL/Hybrid Electric Aicraft System/Hybrid Electric Aicraft Plant/DC//AC Converter/Control open loop1 ==
  Uabc Ref1 : Sin  Amplitude=VL*sqrt(2)  Frequency=2*pi*f  Phase="[0  2*pi/3  -2*pi/3]"  SampleTime=Ts
  g : Outport  VectorParamsAs1DForOutWhenUnconnected=off
  wires:
  Uabc Ref1/1 -> g/1
